simulink model "TFlex_IFITCv2"  (R2018b)
settings: Solver=VariableStepAuto  StartTime=0.0  StopTime=t_end  RelTol=1e-3
values from neighbouring files (symbols this model uses):
  hyp = abs(hyp_sn(1:end-1))    [TFlex_IFITC_init.m]    (also in nlml_I_FITCv2.m = abs(hyp))
  Kuu = SEcov(u,u,hyp) + eye(Mu)*sn2    [nlml_I_FITCv2.m]
  Lu = chol(Kuu,'lower')    [nlml_I_FITCv2.m]
  Mu = 50    [TFlex_IFITC_init.m]    (also in nlml_I_FITCv2.m = length(u))
  Nkeep = 20    [TFlex_IFITC_init.m]
  sn = abs(hyp_sn(end))    [TFlex_IFITC_init.m]
  t_learn = 10    [TFlex_IFITC_init.m]
  t_predict = 15    [TFlex_IFITC_init.m]
  ts = 1/1000    (= 0.001)    [TFlex_IFITC_init.m]
  u_init = u    [TFlex_IFITC_init.m]
undefined symbols (not defined in the file or in its folder): Cogging, DiscIntNeverNeededParam, Hysteresis, I_limit, mu_u, PID, Plant, Reference, SVF, var_u
libraries: simulink x4, dspmtrx3 x3, dspindex x1
settings Model: Creator=wout7  LastModifiedBy=wout7

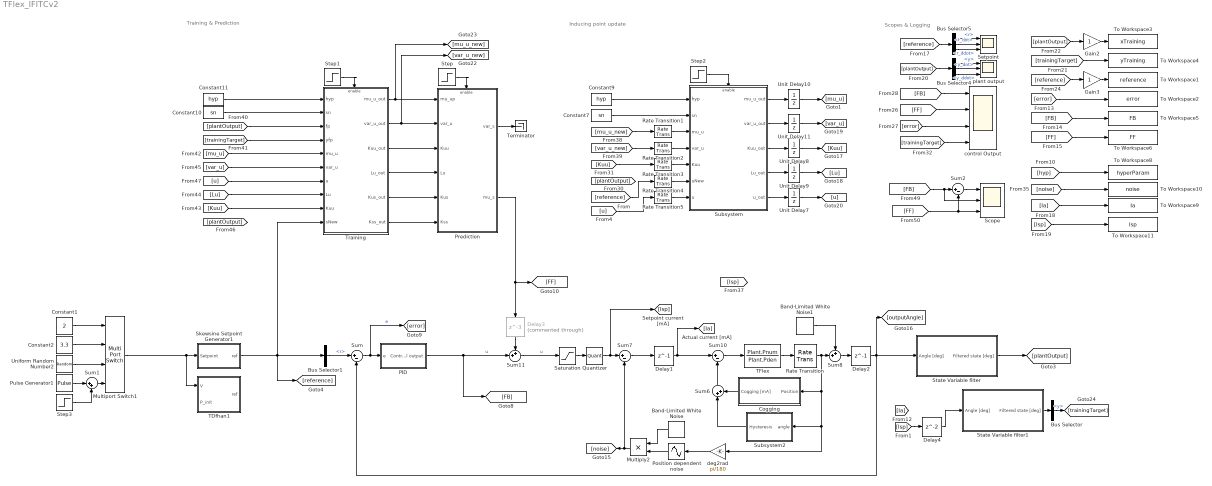
== system TFlex_IFITCv2 ==
  note: Scopes & Logging
  note: Training & Prediction
  note: Inducing point update
  Band-Limited White Noise : simulink/Sources/Band-Limited White Noise  Cov=[1e-3]  Ts=ts  seed=48124
  Band-Limited White Noise1 : simulink/Sources/Band-Limited White Noise  Cov=[1e-13]  Ts=ts  seed=[23341]
  Bus Selector : BusSelector  OutputSignals=y
  Bus Selector1 : BusSelector  OutputSignals=r
  Bus Selector4 : BusSelector  OutputSignals=y,y_dot,y_ddot
  Bus Selector5 : BusSelector  OutputSignals=r,r_dot,r_ddot
  Cogging : Subsystem
  Constant1 : Constant  Value=2  SampleTime=Reference.ts
  Constant10 : Constant  Value=sn  SampleTime=-1
  Constant11 : Constant  Value=hyp  SampleTime=-1
  Constant2 : Constant  Value=3.3  SampleTime=Reference.ts
  Constant7 : Constant  Value=sn  SampleTime=-1
  Constant9 : Constant  Value=hyp  SampleTime=-1
  Delay1 : Delay  DelayLength=1  InitialCondition=0
  Delay2 : Delay  DelayLength=1  InitialCondition=0
  Delay3 : Delay  Commented=through  DelayLength=3  InitialCondition=0
  Delay4 : Delay  InitialCondition=0
  Gain2 : Gain
  Gain3 : Gain
  Multiply2 : Product
  Multiport Switch1 : MultiPortSwitch
  PID : Subsystem
  Position dependent noise : Sin  TimeSource=Use external signal  Bias=2  Frequency=27.7  SampleTime=0
  Prediction : Subsystem
  Pulse Generator1 : DiscretePulseGenerator  Amplitude=2*24  SampleTime=Reference.ts
  Quantizer : Quantizer  QuantizationInterval=1
  Rate Transition : RateTransition  OutPortSampleTime=ts
  Rate Transition{1..5} (5 alike) : RateTransition  OutPortSampleTime=20*ts
  Saturation : Saturate  UpperLimit=I_limit  LowerLimit=-I_limit
  Scope : Scope  NumInputPorts=3
  Setpoint : Scope  NumInputPorts=3
  Skewsine Setpoint Generator1 : Subsystem
  State Variable filter : Subsystem
  State Variable filter1 : Subsystem
  Step : Step  Time=t_predict  SampleTime=ts
  Step1 : Step  Time=t_learn  SampleTime=ts
  Step2 : Step  Time=t_learn  SampleTime=ts
  Step3 : Step  Time=0  After=-24  SampleTime=Reference.ts
  Subsystem : Subsystem
  Subsystem2 : Subsystem
  Sum{,2,7,10} (4 alike) : Sum  Inputs=|+-
  Sum1 : Sum  Inputs=|++
  Sum11 : Sum  Inputs=++|
  Sum6 : Sum  Inputs=|++
  Sum8 : Sum  Inputs=++|
  TDfhan1 : Subsystem
  TFlex : TransferFcn  Numerator=Plant.Pnum  Denominator=Plant.Pden  ContinuousStateAttributes='angle'
  Terminator : Terminator
  To Workspace1 : ToWorkspace  VariableName=reference  SampleTime=-1
  To Workspace10 : ToWorkspace  VariableName=noise  SampleTime=-1
  To Workspace11 : ToWorkspace  VariableName=Isp  SampleTime=-1
  To Workspace2 : ToWorkspace  VariableName=error  SampleTime=-1
  To Workspace3 : ToWorkspace  VariableName=xTraining  SampleTime=-1
  To Workspace4 : ToWorkspace  VariableName=yTraining  SampleTime=-1
  To Workspace5 : ToWorkspace  VariableName=FB  SampleTime=-1
  To Workspace6 : ToWorkspace  VariableName=FF  SampleTime=-1
  To Workspace8 : ToWorkspace  VariableName=hyperParam  SampleTime=-1
  To Workspace9 : ToWorkspace  VariableName=Ia  SampleTime=-1
  Training : Subsystem
  Uniform Random Number2 : UniformRandomNumber  Minimum=-23  Maximum=23  Seed=Reference.seed  SampleTime=Reference.ts
  Unit Delay{7..11} (5 alike) : UnitDelay  SampleTime=-1
  control Output : Scope  NumInputPorts=4
  deg2rad : Gain  Gain=pi/180
  plant output : Scope  NumInputPorts=3
  wires:
  Sum/1 -> PID/1(e), [error]  "e"
  Sum8/1 -> Delay2/1
  Bus Selector1/1 -> Sum/1  "<r>"
  TFlex/1 -> Rate Transition/1
  [reference] -> Gain3/1
  Bus Selector5/2 -> Setpoint/2  "<r_dot>"
  Bus Selector5/1 -> Setpoint/1  "<r>"
  [error] -> To Workspace2/1
  Bus Selector5/3 -> Setpoint/3  "<r_ddot>"
  [FB] -> To Workspace5/1
  [plantOutput] -> Gain2/1
  Gain2/1 -> To Workspace3/1
  [plantOutput] -> Bus Selector4/1
  Gain3/1 -> To Workspace1/1
  Bus Selector4/1 -> plant output/1  "<y>"
  Bus Selector4/3 -> plant output/3  "<y_ddot>"
  [reference] -> Bus Selector5/1
  [trainingTarget] -> To Workspace4/1
  Bus Selector4/2 -> plant output/2  "<y_dot>"
  [FF] -> To Workspace6/1
  [trainingTarget] -> control Output/4
  [FF] -> control Output/2
  [error] -> control Output/3
  [FB] -> control Output/1
  [hyp] -> To Workspace8/1
  Saturation/1 -> Quantizer/1
  PID/1(Control output) -> [FB], Sum11/2  "u"
  State Variable filter/1(Filtered state [deg]) -> [plantOutput]
  Sum11/1 -> Saturation/1  "u"
  Sum10/1 -> TFlex/1
  State Variable filter1/1(Filtered state [deg]) -> Bus Selector/1
  Sum7/1 -> Delay1/1
  Multiply2/1 -> Sum7/2, [noise]
  Rate Transition/1 -> Sum8/2, Cogging/1(Position), deg2rad/1, Subsystem2/1(angle)
  Quantizer/1 -> [Isp], Sum7/1
  Prediction/2(mu_s) -> Delay3/1, [FF]
  Delay3/1 -> Sum11/1
  Band-Limited White Noise/1 -> Multiply2/1
  Position dependent noise/1 -> Multiply2/2
  [noise] -> To Workspace10/1
  [Ia] -> To Workspace9/1
  [Isp] -> To Workspace11/1
  Band-Limited White Noise1/1 -> Sum8/1
  Delay1/1 -> Sum10/1, [Ia]
  [Isp] -> Delay4/1
  Bus Selector/1 -> [trainingTarget]  "<y>"
  Unit Delay10/1 -> [mu_u]
  Unit Delay9/1 -> [Lu]
  Unit Delay7/1 -> [u]
  Unit Delay8/1 -> [Kuu]
  Constant7/1 -> Subsystem/2(sn)
  [mu_u_new] -> Rate Transition1/1
  [var_u_new] -> Rate Transition2/1
  [reference] -> Rate Transition4/1
  Subsystem/1(mu_u_out) -> Unit Delay10/1
  Unit Delay11/1 -> [var_u]
  Subsystem/2(var_u_out) -> Unit Delay11/1
  Subsystem/3(Kuu_out) -> Unit Delay8/1
  Subsystem/4(Lu_out) -> Unit Delay9/1
  Subsystem/5(u_out) -> Unit Delay7/1
  Constant11/1 -> Training/1(hyp)
  Constant10/1 -> Training/2(sn)
  [plantOutput] -> Training/3(fp)
  [trainingTarget] -> Training/4(yfp)
  [mu_u] -> Training/5(mu_u)
  [var_u] -> Training/6(var_u)
  [u] -> Training/7(u)
  [Lu] -> Training/8(Lu)
  [Kuu] -> Training/9(Kuu)
  Training/2(var_u_out) -> [var_u_new], Prediction/2(var_u)
  [FB] -> Scope/2, Sum2/1
  [FF] -> Scope/3, Sum2/2
  Sum2/1 -> Scope/1
  Training/3(Kuu_out) -> Prediction/3(Kuu)
  Training/4(Lu_out) -> Prediction/4(Lu)
  Training/5(Kus_out) -> Prediction/5(Kus)
  Training/6(Kss_out) -> Prediction/6(Kss)
  Prediction/1(var_s) -> Terminator/1
  Training/1(mu_u_out) -> Prediction/1(mu_up), [mu_u_new]
  Step/1 -> Prediction/Enable
  Step2/1 -> Subsystem/Enable
  Step1/1 -> Training/Enable
  [u] -> Rate Transition5/1
  [Kuu] -> Rate Transition3/1
  Constant9/1 -> Subsystem/1(hyp)
  Cogging/1(Cogging [mA]) -> Sum6/2
  Sum6/1 -> Sum10/2
  Subsystem2/1(Hysteresis) -> Sum6/1
  Constant2/1 -> Multiport Switch1/2
  Pulse Generator1/1 -> Sum1/1
  Uniform Random Number2/1 -> Multiport Switch1/3
  Sum1/1 -> Multiport Switch1/4
  Step3/1 -> Sum1/2
  Constant1/1 -> Multiport Switch1/1
  Multiport Switch1/1 -> Skewsine Setpoint Generator1/1(Setpoint), TDfhan1/1(V)
  Skewsine Setpoint Generator1/1(ref) -> Training/10(sNew), Bus Selector1/1, [reference]
  Rate Transition1/1 -> Subsystem/3(mu_u)
  Rate Transition2/1 -> Subsystem/4(var_u)
  Rate Transition3/1 -> Subsystem/5(Kuu)
  Rate Transition4/1 -> Subsystem/6(uNew)
  Rate Transition5/1 -> Subsystem/7(u)
  Delay2/1 -> [outputAngle], State Variable filter/1(Angle [deg]), Sum/2
  deg2rad/1 -> Position dependent noise/1
  Delay4/1 -> State Variable filter1/1(Angle [deg])

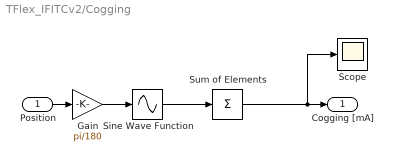
== system TFlex_IFITCv2/Cogging ==
  Position : Inport
  Gain : Gain  Gain=pi/180
  Scope : Scope
  Sine Wave Function : Sin  TimeSource=Use external signal  Amplitude=Cogging.amplitude  Frequency=Cogging.frequency*pi  Phase=Cogging.phase  SampleTime=0
  Sum of Elements : Sum  Inputs=+
  Cogging [mA] : Outport
  wires:
  Sum of Elements/1 -> Scope/1, Cogging [mA]/1
  Sine Wave Function/1 -> Sum of Elements/1
  Position/1 -> Gain/1
  Gain/1 -> Sine Wave Function/1

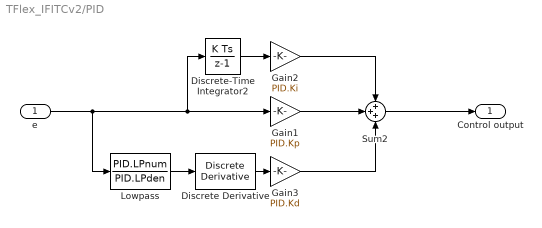
== system TFlex_IFITCv2/PID ==
  e : Inport
  Discrete Derivative : simulink/Discrete/Discrete Derivative  gainval=1.0  ICPrevScaledInput=0.0  OutMin=[]  OutMax=[]  OutDataType=fixdt(1, 16)  OutScaling=2^-10  DoSatur=off
  Discrete-Time Integrator2 : DiscreteIntegrator  SampleTime=-1  ICPrevOutput=DiscIntNeverNeededParam  ICPrevScaledInput=DiscIntNeverNeededParam
  Gain1 : Gain  Gain=PID.Kp
  Gain2 : Gain  Gain=PID.Ki
  Gain3 : Gain  Gain=PID.Kd
  Lowpass : DiscreteTransferFcn  Numerator=PID.LPnum  Denominator=PID.LPden  SampleTime=ts
  Sum2 : Sum  Inputs=3
  Control output : Outport
  wires:
  Discrete-Time Integrator2/1 -> Gain2/1
  Gain1/1 -> Sum2/2
  Gain2/1 -> Sum2/1
  Gain3/1 -> Sum2/3
  Sum2/1 -> Control output/1
  e/1 -> Discrete-Time Integrator2/1, Gain1/1, Lowpass/1
  Lowpass/1 -> Discrete Derivative/1
  Discrete Derivative/1 -> Gain3/1

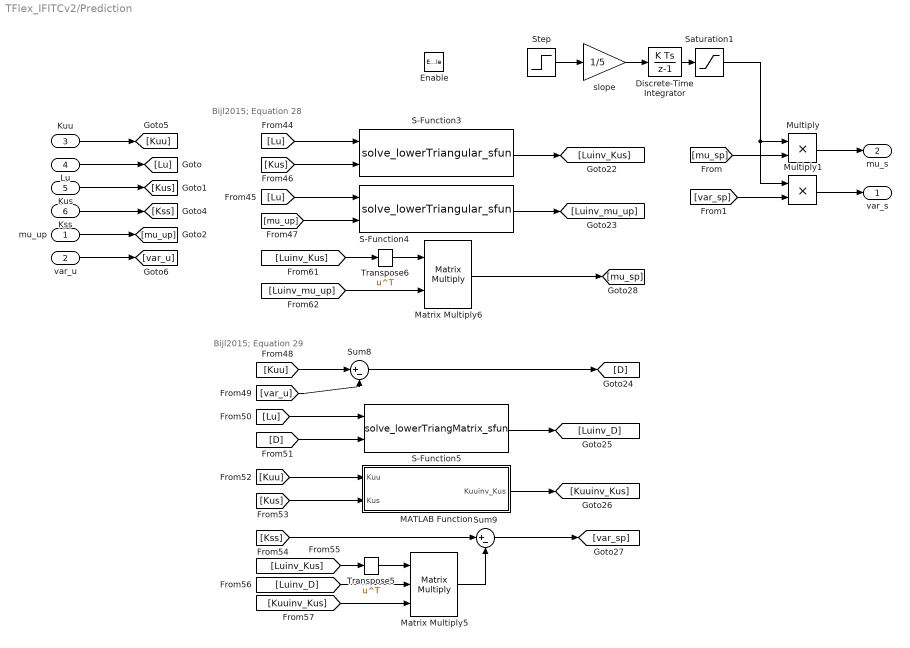
== system TFlex_IFITCv2/Prediction ==
  note: Bijl2015; Equation 29
  note: Bijl2015; Equation 28
  mu_up : Inport
  var_u : Inport  Port=2
  Kuu : Inport  Port=3
  Lu : Inport  Port=4
  Kus : Inport  Port=5
  Kss : Inport  Port=6
  Enable : EnablePort
  Discrete-Time Integrator : DiscreteIntegrator  SampleTime=-1  ICPrevOutput=DiscIntNeverNeededParam  ICPrevScaledInput=DiscIntNeverNeededParam
  MATLAB Function : MATLAB Function  TreatAsAtomicUnit=on
  Matrix Multiply5 : Product  Inputs=3  Multiplication=Matrix(*)
  Matrix Multiply6 : Product  Multiplication=Matrix(*)
  Multiply : Product
  Multiply1 : Product
  S-Function3 : S-Function  FunctionName=solve_lowerTriangular_sfun  Parameters=Nkeep+1  SFunctionDeploymentMode=off  EnableBusSupport=off
  S-Function4 : S-Function  FunctionName=solve_lowerTriangular_sfun  Parameters=Nkeep+1  SFunctionDeploymentMode=off  EnableBusSupport=off
  S-Function5 : S-Function  FunctionName=solve_lowerTriangMatrix_sfun  Parameters=Nkeep+1  SFunctionDeploymentMode=off  EnableBusSupport=off
  Saturation1 : Saturate  UpperLimit=1  LowerLimit=0
  Step : Step  Time=t_predict  SampleTime=0
  Sum8 : Sum  Inputs=|+-
  Sum9 : Sum  Inputs=|+-
  Transpose5 : Math  Operator=transpose  SaturateOnIntegerOverflow=on
  Transpose6 : Math  Operator=transpose  SaturateOnIntegerOverflow=on
  slope : Gain  Gain=1/5
  var_s : Outport
  mu_s : Outport  Port=2
  wires:
  [Luinv_mu_up] -> Matrix Multiply6/2
  S-Function5/1 -> [Luinv_D]
  Transpose5/1 -> Matrix Multiply5/1
  [Luinv_Kus] -> Transpose6/1
  Transpose6/1 -> Matrix Multiply6/1
  [Kus] -> S-Function3/2
  Sum9/1 -> [var_sp]
  Matrix Multiply6/1 -> [mu_sp]
  [Lu] -> S-Function3/1
  [D] -> S-Function5/2
  [Kuu] -> Sum8/1
  [Luinv_Kus] -> Transpose5/1
  [mu_up] -> S-Function4/2
  Sum8/1 -> [D]
  S-Function4/1 -> [Luinv_mu_up]
  S-Function3/1 -> [Luinv_Kus]
  [Kss] -> Sum9/1
  [Lu] -> S-Function5/1
  [Kuu] -> MATLAB Function/1(Kuu)
  [Kus] -> MATLAB Function/2(Kus)
  [Lu] -> S-Function4/1
  [var_u] -> Sum8/2
  Matrix Multiply5/1 -> Sum9/2
  MATLAB Function/1(Kuuinv_Kus) -> [Kuuinv_Kus]
  [Luinv_D] -> Matrix Multiply5/2
  [Kuuinv_Kus] -> Matrix Multiply5/3
  [mu_sp] -> Multiply/2
  [var_sp] -> Multiply1/2
  var_u/1 -> [var_u]
  mu_up/1 -> [mu_up]
  Kss/1 -> [Kss]
  Kus/1 -> [Kus]
  Lu/1 -> [Lu]
  Kuu/1 -> [Kuu]
  Saturation1/1 -> Multiply/1, Multiply1/1
  Step/1 -> slope/1
  slope/1 -> Discrete-Time Integrator/1
  Discrete-Time Integrator/1 -> Saturation1/1
  Multiply/1 -> mu_s/1
  Multiply1/1 -> var_s/1

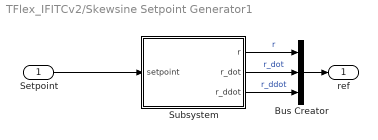
== system TFlex_IFITCv2/Skewsine Setpoint Generator1 ==
  Setpoint : Inport
  Bus Creator : BusCreator  Inputs=3
  Subsystem : Subsystem
  ref : Outport
  wires:
  Subsystem/3(r_ddot) -> Bus Creator/3  "r_ddot"
  Bus Creator/1 -> ref/1
  Subsystem/2(r_dot) -> Bus Creator/2  "r_dot"
  Subsystem/1(r) -> Bus Creator/1  "r"
  Setpoint/1 -> Subsystem/1(setpoint)

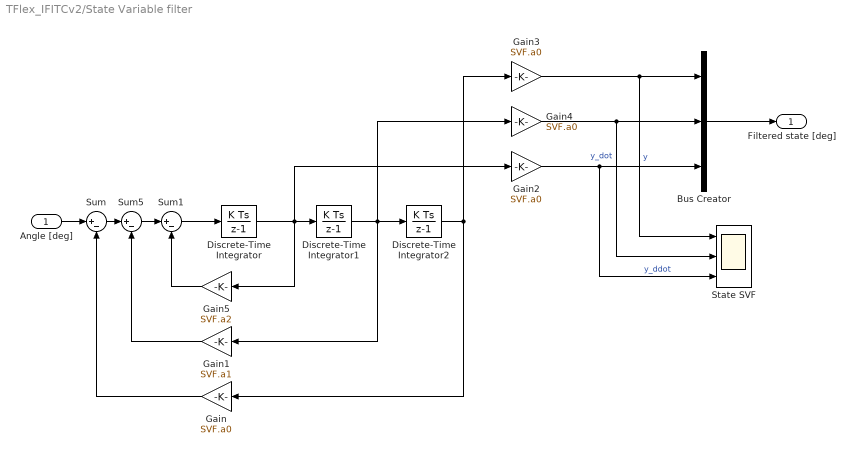
== system TFlex_IFITCv2/State Variable filter ==
  Angle [deg] : Inport
  Bus Creator : BusCreator  Inputs=3
  Discrete-Time Integrator : DiscreteIntegrator  SampleTime=-1  ICPrevOutput=DiscIntNeverNeededParam  ICPrevScaledInput=DiscIntNeverNeededParam
  Discrete-Time Integrator1 : DiscreteIntegrator  SampleTime=-1  ICPrevOutput=DiscIntNeverNeededParam  ICPrevScaledInput=DiscIntNeverNeededParam
  Discrete-Time Integrator2 : DiscreteIntegrator  SampleTime=-1  ICPrevOutput=DiscIntNeverNeededParam  ICPrevScaledInput=DiscIntNeverNeededParam
  Gain{,2..4} (4 alike) : Gain  Gain=SVF.a0
  Gain1 : Gain  Gain=SVF.a1
  Gain5 : Gain  Gain=SVF.a2
  State SVF : Scope  NumInputPorts=3
  Sum : Sum  Inputs=|+-
  Sum1 : Sum  Inputs=|+-
  Sum5 : Sum  Inputs=|+-
  Filtered state [deg] : Outport  SampleTime=ts
  wires:
  Bus Creator/1 -> Filtered state [deg]/1
  Sum1/1 -> Discrete-Time Integrator/1
  Angle [deg]/1 -> Sum/1
  Sum/1 -> Sum5/1
  Gain/1 -> Sum/2
  Gain1/1 -> Sum5/2
  Gain3/1 -> State SVF/1, Bus Creator/1  "y"
  Gain2/1 -> State SVF/3, Bus Creator/3  "y_ddot"
  Gain4/1 -> State SVF/2, Bus Creator/2  "y_dot"
  Gain5/1 -> Sum1/2
  Sum5/1 -> Sum1/1
  Discrete-Time Integrator/1 -> Discrete-Time Integrator1/1, Gain2/1, Gain5/1
  Discrete-Time Integrator1/1 -> Discrete-Time Integrator2/1, Gain4/1, Gain1/1
  Discrete-Time Integrator2/1 -> Gain3/1, Gain/1

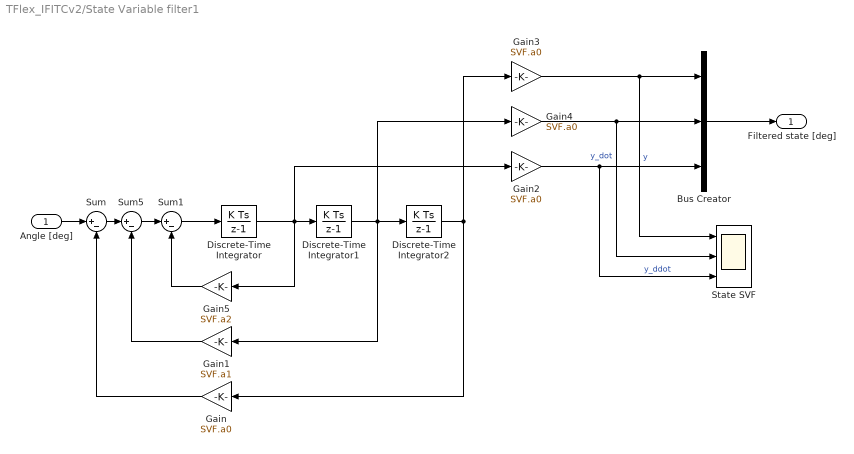
== system TFlex_IFITCv2/State Variable filter1 ==
  Angle [deg] : Inport
  Bus Creator : BusCreator  Inputs=3
  Discrete-Time Integrator : DiscreteIntegrator  SampleTime=-1  ICPrevOutput=DiscIntNeverNeededParam  ICPrevScaledInput=DiscIntNeverNeededParam
  Discrete-Time Integrator1 : DiscreteIntegrator  SampleTime=-1  ICPrevOutput=DiscIntNeverNeededParam  ICPrevScaledInput=DiscIntNeverNeededParam
  Discrete-Time Integrator2 : DiscreteIntegrator  SampleTime=-1  ICPrevOutput=DiscIntNeverNeededParam  ICPrevScaledInput=DiscIntNeverNeededParam
  Gain{,2..4} (4 alike) : Gain  Gain=SVF.a0
  Gain1 : Gain  Gain=SVF.a1
  Gain5 : Gain  Gain=SVF.a2
  State SVF : Scope  NumInputPorts=3
  Sum : Sum  Inputs=|+-
  Sum1 : Sum  Inputs=|+-
  Sum5 : Sum  Inputs=|+-
  Filtered state [deg] : Outport  SampleTime=ts
  wires:
  Bus Creator/1 -> Filtered state [deg]/1
  Sum1/1 -> Discrete-Time Integrator/1
  Angle [deg]/1 -> Sum/1
  Sum/1 -> Sum5/1
  Gain/1 -> Sum/2
  Gain1/1 -> Sum5/2
  Gain3/1 -> State SVF/1, Bus Creator/1  "y"
  Gain2/1 -> State SVF/3, Bus Creator/3  "y_ddot"
  Gain4/1 -> State SVF/2, Bus Creator/2  "y_dot"
  Gain5/1 -> Sum1/2
  Sum5/1 -> Sum1/1
  Discrete-Time Integrator/1 -> Discrete-Time Integrator1/1, Gain2/1, Gain5/1
  Discrete-Time Integrator1/1 -> Discrete-Time Integrator2/1, Gain4/1, Gain1/1
  Discrete-Time Integrator2/1 -> Gain3/1, Gain/1

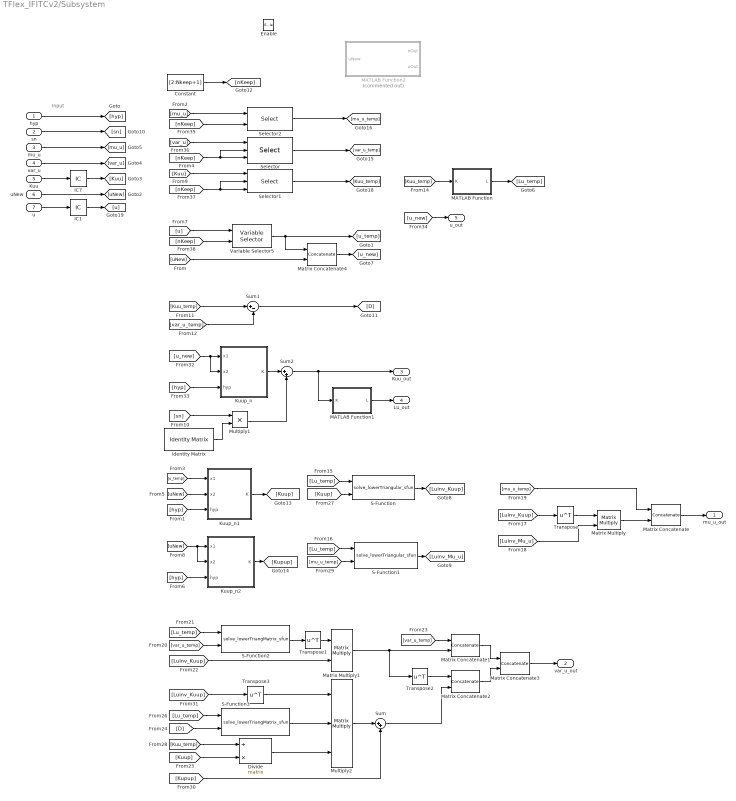
== system TFlex_IFITCv2/Subsystem ==
  note: Input
  hyp : Inport
  sn : Inport  Port=2
  mu_u : Inport  Port=3  PortDimensions=[Nkeep+1,1]
  var_u : Inport  Port=4
  Kuu : Inport  Port=5
  uNew : Inport  Port=6
  u : Inport  Port=7
  Enable : EnablePort
  Constant : Constant  Value=[2:Nkeep+1]
  Divide : Product  Inputs=/*  Multiplication=Matrix(*)
  IC1 : InitialCondition  Value=u
  IC7 : InitialCondition  Value=Kuu
  Identity Matrix : dspmtrx3/Identity Matrix  Inherit=off  N=Nkeep+1  Ts=1  dataType=double  isSigned=on  wordLen=16  udDataType=sfix(16)  fracBitsMode=Best precision  numFracBits=15  OutDataTypeStr=double  LastOutDataTypeStr=double
      settings: SourceProductName=DSP System Toolbox
  Kuup_n : MATLAB Function  TreatAsAtomicUnit=on
  Kuup_n1 : MATLAB Function  TreatAsAtomicUnit=on
  Kuup_n2 : MATLAB Function  TreatAsAtomicUnit=on
  MATLAB Function : MATLAB Function  TreatAsAtomicUnit=on
  MATLAB Function1 : MATLAB Function  TreatAsAtomicUnit=on
  MATLAB Function2 : MATLAB Function  Commented=on  TreatAsAtomicUnit=on
  Matrix Concatenate : Concatenate  Mode=Multidimensional array
  Matrix Concatenate1 : Concatenate  Mode=Multidimensional array  ConcatenateDimension=2
  Matrix Concatenate2 : Concatenate  Mode=Multidimensional array  ConcatenateDimension=2
  Matrix Concatenate3 : Concatenate  Mode=Multidimensional array
  Matrix Concatenate4 : Concatenate  Mode=Multidimensional array
  Matrix Multiply : Product  Multiplication=Matrix(*)
  Matrix Multiply1 : Product  Multiplication=Matrix(*)
  Multiply1 : Product
  Multiply2 : Product  Inputs=3  Multiplication=Matrix(*)
  S-Function : S-Function  FunctionName=solve_lowerTriangular_sfun  Parameters=Nkeep  SFunctionDeploymentMode=off  EnableBusSupport=off
  S-Function1 : S-Function  FunctionName=solve_lowerTriangular_sfun  Parameters=Nkeep  SFunctionDeploymentMode=off  EnableBusSupport=off
  S-Function2 : S-Function  FunctionName=solve_lowerTriangMatrix_sfun  Parameters=Nkeep  SFunctionDeploymentMode=off  EnableBusSupport=off
  S-Function3 : S-Function  FunctionName=solve_lowerTriangMatrix_sfun  Parameters=Nkeep  SFunctionDeploymentMode=off  EnableBusSupport=off
  Selector : Selector  NumberOfDimensions=2  InputPortWidth=3  IndexOptions=Index vector (port),Index vector (port)  Indices=[1 3],1  OutputSizes=1,1
  Selector1 : Selector  NumberOfDimensions=2  InputPortWidth=3  IndexOptions=Index vector (port),Index vector (port)  Indices=[1 3],1  OutputSizes=1,1
  Selector2 : Selector  InputPortWidth=Nkeep+1  IndexOptions=Index vector (port)  Indices=[1 3]  OutputSizes=1
  Sum : Sum  Inputs=|++
  Sum1 : Sum  Inputs=|+-
  Sum2 : Sum  Inputs=|++
  Transpose{,1..3} (4 alike) : Math  Operator=transpose  SaturateOnIntegerOverflow=on
  Variable Selector5 : dspindex/Variable Selector  NumInputs=1  rowsOrCols=Rows  IdxMode=Variable  Elements=[1 3]  ZerOneIdxMode=One-based  errmode=Clip Index  FillMode=off  FillValues=0
  mu_u_out : Outport
  var_u_out : Outport  Port=2
  Kuu_out : Outport  Port=3
  Lu_out : Outport  Port=4
  u_out : Outport  Port=5  PortDimensions=[Mu,3]
  wires:
  hyp/1 -> [hyp]
  [hyp] -> Kuup_n1/3(hyp)
  [u_temp] -> Kuup_n1/1(x1)
  [uNew] -> Kuup_n1/2(x2)
  [uNew] -> Kuup_n2/2(x2), Kuup_n2/1(x1)
  [hyp] -> Kuup_n2/3(hyp)
  mu_u/1 -> [mu_u]
  [Lu_temp] -> S-Function/1
  S-Function/1 -> [Luinv_Kuup]
  S-Function1/1 -> [Luinv_Mu_u]
  [Lu_temp] -> S-Function1/1
  Kuup_n2/1(K) -> [Kupup]
  [Luinv_Kuup] -> Transpose/1
  Transpose/1 -> Matrix Multiply/1
  [Luinv_Mu_u] -> Matrix Multiply/2
  Matrix Multiply/1 -> Matrix Concatenate/2
  [mu_u_temp] -> Matrix Concatenate/1
  Matrix Concatenate/1 -> mu_u_out/1
  [var_u_temp] -> S-Function2/2
  [Lu_temp] -> S-Function2/1
  S-Function2/1 -> Transpose1/1
  Transpose1/1 -> Matrix Multiply1/1
  [Luinv_Kuup] -> Matrix Multiply1/2
  Matrix Multiply1/1 -> Transpose2/1, Matrix Concatenate1/2
  [var_u_temp] -> Matrix Concatenate1/1
  Transpose2/1 -> Matrix Concatenate2/1
  Matrix Concatenate1/1 -> Matrix Concatenate3/1
  Matrix Concatenate2/1 -> Matrix Concatenate3/2
  [D] -> S-Function3/2
  [Lu_temp] -> S-Function3/1
  [Kuup] -> Divide/2
  [Kuu_temp] -> Divide/1
  Divide/1 -> Multiply2/3
  Kuup_n1/1(K) -> [Kuup]
  [Kuup] -> S-Function/2
  [mu_u_temp] -> S-Function1/2
  [Luinv_Kuup] -> Transpose3/1
  Transpose3/1 -> Multiply2/1
  Multiply2/1 -> Sum/1
  [Kupup] -> Sum/2
  Sum/1 -> Matrix Concatenate2/2
  Matrix Concatenate3/1 -> var_u_out/1
  Identity Matrix/1 -> Multiply1/2
  [sn] -> Multiply1/1
  [u_new] -> Kuup_n/2(x2), Kuup_n/1(x1)
  [hyp] -> Kuup_n/3(hyp)
  Multiply1/1 -> Sum2/2
  Kuup_n/1(K) -> Sum2/1
  Sum2/1 -> Kuu_out/1, MATLAB Function1/1(K)
  MATLAB Function1/1(L) -> Lu_out/1
  [u_new] -> u_out/1
  S-Function3/1 -> Multiply2/2
  Variable Selector5/1 -> [u_temp], Matrix Concatenate4/1
  [mu_u] -> Selector2/1
  Selector2/1 -> [mu_u_temp]
  sn/1 -> [sn]
  [Kuu_temp] -> Sum1/1
  [var_u_temp] -> Sum1/2
  Sum1/1 -> [D]
  [Kuu_temp] -> MATLAB Function/1(K)
  MATLAB Function/1(L) -> [Lu_temp]
  Kuu/1 -> IC7/1
  [nKeep] -> Selector2/2
  [nKeep] -> Selector/2, Selector/3
  [Kuu] -> Selector1/1
  [nKeep] -> Variable Selector5/2
  [nKeep] -> Selector1/2, Selector1/3
  Selector1/1 -> [Kuu_temp]
  uNew/1 -> [uNew]
  [u] -> Variable Selector5/1
  u/1 -> IC1/1
  [var_u] -> Selector/1
  Selector/1 -> [var_u_temp]
  var_u/1 -> [var_u]
  [uNew] -> Matrix Concatenate4/2
  Matrix Concatenate4/1 -> [u_new]
  IC1/1 -> [u]
  IC7/1 -> [Kuu]
  Constant/1 -> [nKeep]

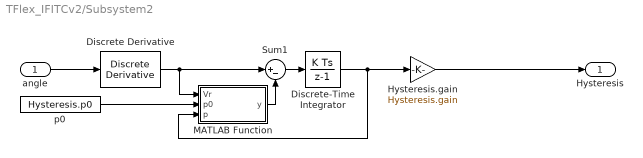
== system TFlex_IFITCv2/Subsystem2 ==
  angle : Inport
  Discrete Derivative : simulink/Discrete/Discrete Derivative  gainval=1.0  ICPrevScaledInput=0.0  OutMin=[]  OutMax=[]  OutDataType=fixdt(1, 16)  OutScaling=2^-10  DoSatur=off
  Discrete-Time Integrator : DiscreteIntegrator  SampleTime=-1  ICPrevOutput=DiscIntNeverNeededParam  ICPrevScaledInput=DiscIntNeverNeededParam
  Hysteresis.gain : Gain  Gain=Hysteresis.gain
  MATLAB Function : MATLAB Function  TreatAsAtomicUnit=on
  Sum1 : Sum  Inputs=|+-
  p0 : Constant  Value=Hysteresis.p0
  Hysteresis : Outport
  wires:
  MATLAB Function/1(y) -> Sum1/2
  angle/1 -> Discrete Derivative/1
  Sum1/1 -> Discrete-Time Integrator/1
  Discrete Derivative/1 -> Sum1/1, MATLAB Function/1(Vr)
  Discrete-Time Integrator/1 -> MATLAB Function/3(p), Hysteresis.gain/1
  Hysteresis.gain/1 -> Hysteresis/1
  p0/1 -> MATLAB Function/2(p0)

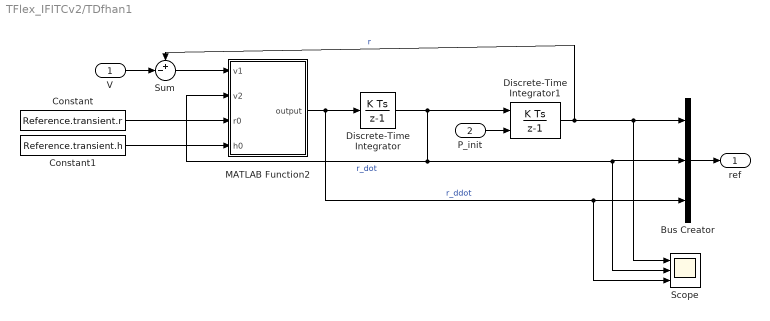
== system TFlex_IFITCv2/TDfhan1 ==
  V : Inport
  P_init : Inport  Port=2
  Bus Creator : BusCreator  Inputs=3
  Constant : Constant  Value=Reference.transient.r  SampleTime=ts
  Constant1 : Constant  Value=Reference.transient.h  SampleTime=ts
  Discrete-Time Integrator : DiscreteIntegrator  gainval=1  SampleTime=ts  ICPrevOutput=DiscIntNeverNeededParam  ICPrevScaledInput=DiscIntNeverNeededParam
  Discrete-Time Integrator1 : DiscreteIntegrator  gainval=1  InitialConditionSource=external  InitialCondition=-24  SampleTime=ts  ICPrevOutput=DiscIntNeverNeededParam  ICPrevScaledInput=DiscIntNeverNeededParam
  MATLAB Function2 : MATLAB Function  TreatAsAtomicUnit=on
  Scope : Scope  NumInputPorts=3
  Sum : Sum  Inputs=+-|
  ref : Outport
  wires:
  Sum/1 -> MATLAB Function2/1(v1)
  V/1 -> Sum/2
  Constant/1 -> MATLAB Function2/3(r0)
  Constant1/1 -> MATLAB Function2/4(h0)
  P_init/1 -> Discrete-Time Integrator1/2
  Discrete-Time Integrator1/1 -> Sum/1, Scope/1, Bus Creator/1  "r"
  Discrete-Time Integrator/1 -> Discrete-Time Integrator1/1, Scope/2, Bus Creator/2, MATLAB Function2/2(v2)  "r_dot"
  Bus Creator/1 -> ref/1
  MATLAB Function2/1(output) -> Scope/3, Bus Creator/3, Discrete-Time Integrator/1  "r_ddot"

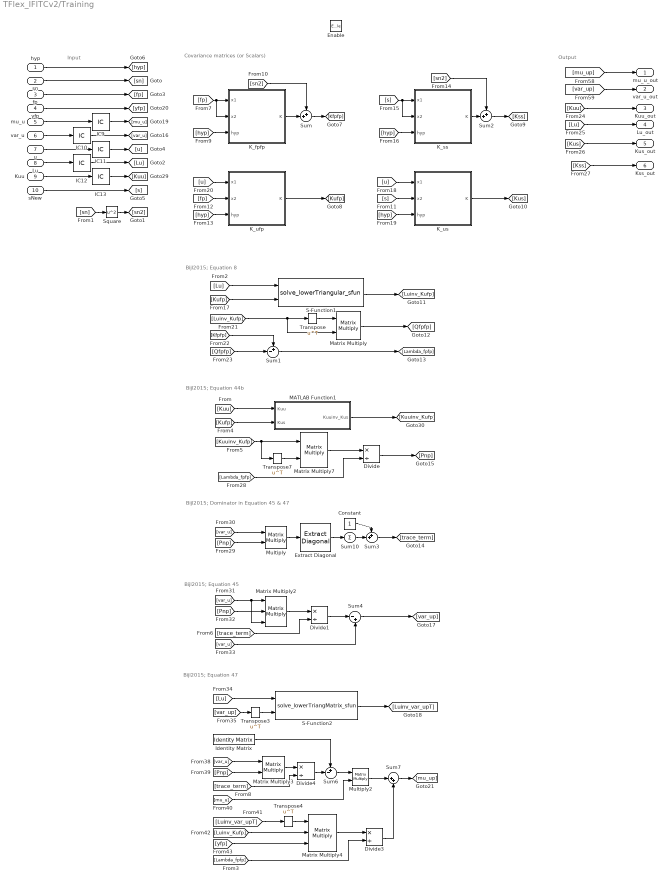
== system TFlex_IFITCv2/Training ==
  note: Output
  note: Input
  note: Covariance matrices (or Scalars)
  note: Bijl2015; Equation 47
  note: Bijl2015; Dominator in Equation 45 & 47
  note: Bijl2015; Equation 45
  note: Bijl2015; Equation 44b
  note: Bijl2015; Equation 8
  hyp : Inport
  sn : Inport  Port=2
  fp : Inport  Port=3
  yfp : Inport  Port=4
  mu_u : Inport  Port=5
  var_u : Inport  Port=6
  u : Inport  Port=7
  Lu : Inport  Port=8
  Kuu : Inport  Port=9
  sNew : Inport  Port=10  PortDimensions=[1,3]
  Enable : EnablePort
  Constant : Constant
  Divide{,1,3..4} (4 alike) : Product  Inputs=*/
  Extract Diagonal : dspmtrx3/Extract Diagonal
      settings: SourceProductName=DSP System Toolbox  SourceProductBaseCode=DS
  IC10 : InitialCondition  Value=var_u
  IC11 : InitialCondition  Value=u
  IC12 : InitialCondition  Value=Lu
  IC13 : InitialCondition  Value=Kuu
  IC9 : InitialCondition  Value=mu_u
  Identity Matrix : dspmtrx3/Identity Matrix  Inherit=off  N=Nkeep+1  Ts=1  dataType=double  isSigned=on  wordLen=16  udDataType=sfix(16)  fracBitsMode=Best precision  numFracBits=15  OutDataTypeStr=double  LastOutDataTypeStr=double
      settings: SourceProductName=DSP System Toolbox
  "K_fpfp " : MATLAB Function  TreatAsAtomicUnit=on
  K_ss : MATLAB Function  TreatAsAtomicUnit=on
  K_ufp : MATLAB Function  TreatAsAtomicUnit=on
  K_us : MATLAB Function  TreatAsAtomicUnit=on
  MATLAB Function1 : MATLAB Function  TreatAsAtomicUnit=on
  Matrix Multiply : Product  Multiplication=Matrix(*)
  Matrix Multiply2 : Product  Inputs=3  Multiplication=Matrix(*)
  Matrix Multiply3 : Product  Multiplication=Matrix(*)
  Matrix Multiply4 : Product  Inputs=3  Multiplication=Matrix(*)
  Matrix Multiply7 : Product  Multiplication=Matrix(*)
  Multiply : Product  Multiplication=Matrix(*)
  Multiply2 : Product  Multiplication=Matrix(*)
  S-Function1 : S-Function  FunctionName=solve_lowerTriangular_sfun  Parameters=Nkeep+1  SFunctionDeploymentMode=off  EnableBusSupport=off
  S-Function2 : S-Function  FunctionName=solve_lowerTriangMatrix_sfun  Parameters=Nkeep+1  SFunctionDeploymentMode=off  EnableBusSupport=off
  Square : Math  Operator=square  SaturateOnIntegerOverflow=on
  Sum : Sum  Inputs=++|
  Sum1 : Sum  Inputs=+-|
  Sum10 : Sum  Inputs=+
  Sum2 : Sum  Inputs=++|
  Sum3 : Sum  Inputs=++|
  Sum4 : Sum  Inputs=|-+
  Sum6 : Sum  Inputs=+-|
  Sum7 : Sum  Inputs=|++
  Transpose{,3..4,7} (4 alike) : Math  Operator=transpose  SaturateOnIntegerOverflow=on
  mu_u_out : Outport
  var_u_out : Outport  Port=2
  Kuu_out : Outport  Port=3
  Lu_out : Outport  Port=4
  Kus_out : Outport  Port=5
  Kss_out : Outport  Port=6
  wires:
  yfp/1 -> [yfp]
  sn/1 -> [sn]
  Lu/1 -> IC12/1
  var_u/1 -> IC10/1
  [sn] -> Square/1
  Square/1 -> [sn2]
  fp/1 -> [fp]
  u/1 -> IC11/1
  sNew/1 -> [s]
  [fp] -> "K_fpfp "/2(x2), "K_fpfp "/1(x1)
  hyp/1 -> [hyp]
  [hyp] -> "K_fpfp "/3(hyp)
  "K_fpfp "/1(K) -> Sum/2
  [sn2] -> Sum/1
  Sum/1 -> [Kfpfp]
  [fp] -> K_ufp/2(x2)
  [hyp] -> K_ufp/3(hyp)
  K_ufp/1(K) -> [Kufp]
  Sum2/1 -> [Kss]
  [s] -> K_ss/1(x1), K_ss/2(x2)
  [hyp] -> K_ss/3(hyp)
  [sn2] -> Sum2/1
  K_ss/1(K) -> Sum2/2
  K_us/1(K) -> [Kus]
  [u] -> K_us/1(x1)
  [hyp] -> K_us/3(hyp)
  [u] -> K_ufp/1(x1)
  [s] -> K_us/2(x2)
  S-Function1/1 -> [Luinv_Kufp]
  [Lu] -> S-Function1/1
  [Kufp] -> S-Function1/2
  Transpose/1 -> Matrix Multiply/1
  [Luinv_Kufp] -> Transpose/1, Matrix Multiply/2
  Matrix Multiply/1 -> [Qfpfp]
  Sum1/1 -> [Lambda_fpfp]
  [Kfpfp] -> Sum1/1
  [Qfpfp] -> Sum1/2
  [Pnp] -> Matrix Multiply2/2
  Matrix Multiply2/1 -> Divide1/1
  [trace_term] -> Divide1/2
  Sum4/1 -> [var_up]
  S-Function2/1 -> [Luinv_var_upT]
  [Lu] -> S-Function2/1
  [var_up] -> Transpose3/1
  Transpose3/1 -> S-Function2/2
  [var_u] -> Matrix Multiply3/1
  [Pnp] -> Matrix Multiply3/2
  mu_u/1 -> IC9/1
  Identity Matrix/1 -> Sum6/1
  [mu_u] -> Multiply2/2
  Transpose4/1 -> Matrix Multiply4/1
  [Luinv_var_upT] -> Transpose4/1
  [Luinv_Kufp] -> Matrix Multiply4/2
  [yfp] -> Matrix Multiply4/3
  Multiply2/1 -> Sum7/1
  Divide3/1 -> Sum7/2
  Sum7/1 -> [mu_up]
  [mu_up] -> mu_u_out/1
  [var_up] -> var_u_out/1
  Kuu/1 -> IC13/1
  Matrix Multiply4/1 -> Divide3/1
  [Lambda_fpfp] -> Divide3/2
  Sum6/1 -> Multiply2/1
  Matrix Multiply3/1 -> Divide4/1
  Divide4/1 -> Sum6/2
  [Kuu] -> MATLAB Function1/1(Kuu)
  [Kufp] -> MATLAB Function1/2(Kus)
  MATLAB Function1/1(Kuuinv_Kus) -> [Kuuinv_Kufp]
  [Kuuinv_Kufp] -> Transpose7/1, Matrix Multiply7/1
  Transpose7/1 -> Matrix Multiply7/2
  Matrix Multiply7/1 -> Divide/1
  Divide/1 -> [Pnp]
  [Lambda_fpfp] -> Divide/2
  [var_u] -> Matrix Multiply2/3, Matrix Multiply2/1
  Divide1/1 -> Sum4/1
  [var_u] -> Sum4/2
  Sum10/1 -> Sum3/2
  Constant/1 -> Sum3/1
  [Pnp] -> Multiply/2
  Multiply/1 -> Extract Diagonal/1
  [var_u] -> Multiply/1
  Extract Diagonal/1 -> Sum10/1
  Sum3/1 -> [trace_term]
  [trace_term] -> Divide4/2
  [Kuu] -> Kuu_out/1
  [Lu] -> Lu_out/1
  [Kus] -> Kus_out/1
  [Kss] -> Kss_out/1
  IC13/1 -> [Kuu]
  IC9/1 -> [mu_u]
  IC10/1 -> [var_u]
  IC11/1 -> [u]
  IC12/1 -> [Lu]

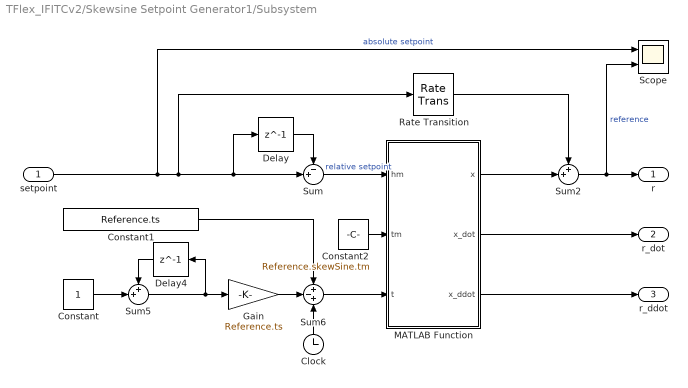
== system TFlex_IFITCv2/Skewsine Setpoint Generator1/Subsystem ==
  setpoint : Inport
  Clock : Clock
      settings: Decimation=100
  Constant : Constant  SampleTime=Reference.ts
  Constant1 : Constant  Value=Reference.ts  SampleTime=Reference.ts
  Constant2 : Constant  Value=Reference.skewSine.tm  SampleTime=Reference.ts
  Delay : Delay  DelayLength=1  InitialCondition=0  SampleTime=Reference.ts
  Delay4 : Delay  DelayLength=1  InitialCondition=0  SampleTime=Reference.ts
  Gain : Gain  Gain=Reference.ts
  MATLAB Function : MATLAB Function  TreatAsAtomicUnit=on
  Rate Transition : RateTransition  OutPortSampleTime=ts
  Scope : Scope  NumInputPorts=2
  Sum : Sum  Inputs=-+|
  Sum2 : Sum  Inputs=++|
  Sum5 : Sum  Inputs=++|
  Sum6 : Sum  Inputs=+-+
  r : Outport
  r_dot : Outport  Port=2
  r_ddot : Outport  Port=3
  wires:
  Delay4/1 -> Sum5/1
  Sum2/1 -> r/1, Scope/2  "reference"
  Sum5/1 -> Delay4/1, Gain/1
  Constant/1 -> Sum5/2
  MATLAB Function/3(x_ddot) -> r_ddot/1
  Clock/1 -> Sum6/3
  Delay/1 -> Sum/1
  Gain/1 -> Sum6/2
  Constant1/1 -> Sum6/1
  MATLAB Function/2(x_dot) -> r_dot/1
  Sum/1 -> MATLAB Function/1(hm)  "relative setpoint"
  Constant2/1 -> MATLAB Function/2(tm)
  Sum6/1 -> MATLAB Function/3(t)
  MATLAB Function/1(x) -> Sum2/2
  setpoint/1 -> Scope/1, Rate Transition/1, Delay/1, Sum/2  "absolute setpoint"
  Rate Transition/1 -> Sum2/1

== matlab function TFlex_IFITCv2/Subsystem/Kuup_n1 ==
  data: x1 input; K output size=[Nkeep,1]; x2 input; hyp input
function K = SquaredExpCov(x1,x2,hyp) %#codegen
coder.extrinsic('SEcov');
n = size(x1,1);
K = double(zeros(n,1));
K = SEcov(x1,x2,hyp);
end

== matlab function TFlex_IFITCv2/Subsystem2/MATLAB Function ==
  data: Vr input; p0 input; y output; p input
function y = fcn(Vr,p0,p)
if Vr>0 && p>=p0
    y = Vr;
elseif Vr<0 && p<=-p0
    y = Vr;
else
    y = 0;
end

== matlab function TFlex_IFITCv2/Prediction/MATLAB Function ==
  data: Kuu input; Kuuinv_Kus output; Kus input
function Kuuinv_Kus = linSolve(Kuu,Kus)
Kuuinv_Kus = Kuu\Kus;

== matlab function TFlex_IFITCv2/Subsystem/Kuup_n2 ==
  data: x1 input; K output size=[1,1]; x2 input; hyp input
function K = SquaredExpCov(x1,x2,hyp) %#codegen
coder.extrinsic('SEcov');
K = double(1);
K = SEcov(x1,x2,hyp);
end

== matlab function TFlex_IFITCv2/Subsystem/MATLAB Function ==
  data: K input; L output
function L = calcChol(K)
L = chol(K,'lower');

== matlab function TFlex_IFITCv2/Training/K_fpfp  ==
  data: x1 input size=[1,3]; K output size=[1,1]; x2 input size=[1,3]; hyp input
function K = SquaredExpCov(x1,x2,hyp) %#codegen
coder.extrinsic('SEcov');
n = size(x1,1);
K = double(zeros(n,1));
K = SEcov(x1,x2,hyp);
end

== matlab function TFlex_IFITCv2/Subsystem/Kuup_n ==
  data: x1 input; K output size=[Nkeep+1,Nkeep+1]; x2 input; hyp input
function K = SquaredExpCov(x1,x2,hyp) %#codegen
coder.extrinsic('SEcov');
n = size(x1,1);
K = double(zeros(n));
K = SEcov(x1,x2,hyp);
end

== matlab function TFlex_IFITCv2/Training/K_ufp ==
  data: x1 input; K output size=[Nkeep+1,1]; x2 input; hyp input
function K = SquaredExpCov(x1,x2,hyp) %#codegen
coder.extrinsic('SEcov');
n = size(x1,1);
K = double(zeros(n,1));
K = SEcov(x1,x2,hyp);
end

== matlab function TFlex_IFITCv2/Training/K_ss ==
  data: x1 input; K output; x2 input; hyp input
function K = SquaredExpCov(x1,x2,hyp) %#codegen
coder.extrinsic('SEcov');
n = size(x1,1);
K = double(zeros(n,1));
K = SEcov(x1,x2,hyp);
end

== matlab function TFlex_IFITCv2/Training/K_us ==
  data: x1 input; K output size=[Nkeep+1,1]; x2 input; hyp input
function K = SquaredExpCov(x1,x2,hyp) %#codegen
coder.extrinsic('SEcov');
n = size(x1,1);
K = double(zeros(n,1));
K = SEcov(x1,x2,hyp);
end

== matlab function TFlex_IFITCv2/Subsystem/MATLAB Function2 ==
  data: uNew input; nOut output size=1; uOut output size=[Nkeep+1,3]; u_init parameter; Nkeep parameter
function [nOut, uOut]  = inducingPoints(uNew,u_init, Nkeep)
persistent u n NORM minNorm
%% Initialize latin hypercube
if isempty(u)
    u = double(u_init);
    n = double(1);
    NORM = double(-(ones(Nkeep+1,Nkeep+1)-eye(Nkeep+1)));    %Initial matrix with norms
    minNorm = double(0);    % Min. norm in set of inducing points
end
%
uNew = double(uNew);

%% Update latin hypercube
one = ones(Nkeep+1,1);
XNEW = [uNew(1,1).*one, uNew(1,2).*one, uNew(1,3).*one];
size(XNEW)
%xNew = (xTrain(:,sample)' - mu_X) ./ sig_X; % New sample
d_new = sqrt(sum((u-XNEW ).^2,2));      % Norms between new sample and inducing points
d_min = min(d_new);                 % Minimal norm for new sample
if (d_min > minNorm)
    d_new(n)  = 0;          % For zero on diagonal
    NORM_temp = NORM;
    
    NORM_temp(n,:) = d_new';     %
    NORM_temp(:,n) = d_new;      %
    NORM = NORM_temp;
    u_copy    = u;
    u_copy(n,:) = uNew;             % Replace inducing point with new sample
    u = u_copy;
    replaceU  = true;
    nOut      = n;
    %Find new min. norm between inducing points
    [minNormTemp nTemp] = min(min(NORM+eye(Nkeep+1)*1e6));
    n = nTemp;
    minNorm = minNormTemp;
end
%}
uOut  = u;
nOut  = n;
%nOut = [2:Nkeep+1]';

== matlab function TFlex_IFITCv2/Training/MATLAB Function1 ==
  data: Kuu input; Kuuinv_Kus output size=[Nkeep+1,1]; Kus input
function Kuuinv_Kus = linSolve(Kuu,Kus)
Kuuinv_Kus = Kuu\Kus;

== matlab function TFlex_IFITCv2/Skewsine Setpoint Generator1/Subsystem/MATLAB Function ==
  settings: updateMethod=DISCRETE  sampleTime=ts
  data: hm input; x output; tm input; t input; x_dot output; x_ddot output
function [x,x_dot,x_ddot] = skewSine(hm,tm,t)

if (t>=0) && (t<=tm)
    x      = hm/tm*t - hm/(2*pi)*sin(2*pi/tm*t);
    x_dot  = hm/tm - hm/tm*cos(2*pi/tm*t);
    x_ddot = 2*pi*hm/(tm^2)*sin(2*pi/tm*t);
else
    x      = hm;
    x_dot  = 0;
    x_ddot = 0;
end

== matlab function TFlex_IFITCv2/TDfhan1/MATLAB Function2 ==
  data: v1 input; output output; v2 input; r0 input; h0 input
function output = Fhan(v1,v2,r0, h0)
d = h0^2*r0;
a0 = h0*v2;
y = v1 + a0;
a1 = sqrt(d*(d+8*abs(y)));
a2 = a0 + sign(y)*(a1-d)/2;
sy = (sign(y+d)-sign(y-d))/2;
a = (a0+y-a2)*sy +a2;
sa = (sign(a+d)-sign(a-d))/2;
output = -r0 *(a/d -sign(a) )*sa - r0*sign(a);

== matlab function TFlex_IFITCv2/Subsystem/MATLAB Function1 ==
  data: K input; L output
function L = calcChol(K)
L = chol(K,'lower');
